simulink library "aerolib_blown_block"  (R2022b)
settings: Solver=ode45  StartTime=0.0  StopTime=10.0  RelTol=1e-3
PostLoadFcn:
  | load_system('aerolibv1')
  | setsysloc('aerolibv1')
libraries: aerolibadynsys x6, sharedutil x1
Description:
  | Aerospace Blockset Library: Aerodynamic library
settings Model: FPTRunName=Active  Creator=The MathWorks, Inc.  LastModifiedBy=olinw
settings SolverCC: AlgebraicLoopSolver=TrustRegion  MaxZcPerStep=1
settings DataIOCC: LimitDataPoints=on  SaveFormat=Array  SignalLoggingSaveFormat=ModelDataLogs  ReturnWorkspaceOutputs=off
settings OptimizationCC: BlockReduction=off  BooleanDataType=off  ExpressionDepthLimit=2147483647  EfficientMapNaN2IntZero=off  LifeSpan=inf
settings DebuggingCC: SaveWithParameterizedLinksMsg=none  UnderspecifiedInitializationDetection=Classic  MergeDetectMultiDrivingBlocksExec=none  SignalResolutionControl=TryResolveAllWithWarning  FcnCallInpInsideContextMsg=warning  UnconnectedInputMsg=warning  UnconnectedOutputMsg=warning  UnconnectedLineMsg=warning  AllowSymbolicDim=off  StateNameClashWarn=warning  SFUnexpectedBacktrackingDiag=warning  SFNoUnconditionalDefaultTransitionDiag=warning  SFExecutionAtInitializationDiag=none  SFMachineParentedDataDiag=warning  ArithmeticOperatorsInVariantConditions=warning
settings HardwareCC: ProdBitPerPointer=32  ProdLargestAtomicFloat=None  ProdIntDivRoundTo=Undefined  ProdEndianess=Unspecified  ProdWordSize=32  ProdHWDeviceType=32-bit Generic  TargetUnknown=on
settings ModelReferenceCC: EnableRefExpFcnMdlSchedulingChecks=on  PropagateSignalLabelsOutOfModel=off
settings SFSimCC: SimUseLocalCustomCode=off  CustomCodeUndefinedFunction=UseInterfaceOnly
settings RTWCC: RTWUseLocalCustomCode=off  DLArmComputeVersion=19.05
settings CodeAppCC: StateflowObjectComments=on
settings GRTTargetCC: TargetLangStandard=C89/C90 (ANSI)  CombineOutputUpdateFcns=off  GRTInterface=on
settings ConfigComp: CovMetricSettings=dw  CovSaveCumulativeToWorkspaceVar=on  CovSaveSingleToWorkspaceVar=on  CovExternalEMLEnable=off

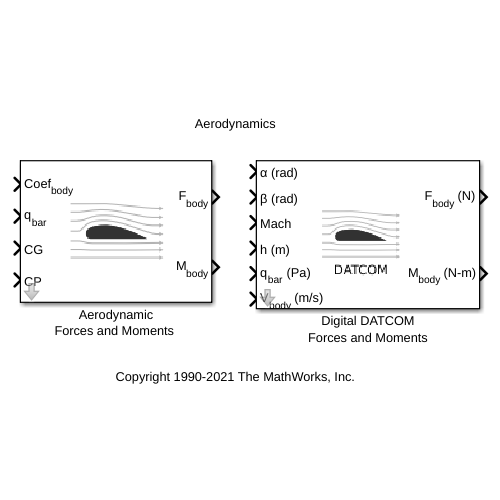
[thumbnail: Simulink's stored preview of the top-level diagram]
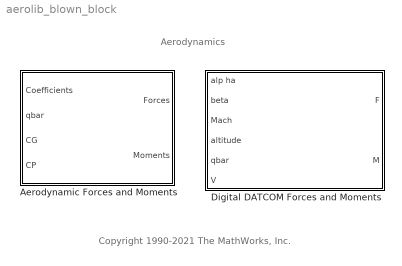
== system aerolib_blown_block ==
  note: Aerodynamics
  note: Copyright 1990-2021 The MathWorks, Inc.
  "Aerodynamic Forces and Moments " : Subsystem  BlockKeywords=__PRM__SERIALIZED__DATA__:Aerodynamic Forces and Moments,aerodynamics,aerodynamic coefficients  mask(Aerodynamic Forces and Moments){inputAxes=Body, outputForceAxes=Body, outputMomentAxes=Body, S=1, b=1, cbar=1}
      mask prompts: inputAxes "aeroblks:aeroblkadyn:blockAerodynamicForcesandMomentsParamInputaxes"; outputForceAxes "aeroblks:aeroblkadyn:blockAerodynamicForcesandMomentsParamForceaxes"; outputMomentAxes "aeroblks:aeroblkadyn:blockAerodynamicForcesandMomentsParamMomentaxes"; S "aeroblks:aeroblkadyn:blockAerodynamicForcesandMomentsParamReferencearea"; b "aeroblks:aeroblkadyn:blockAerodynamicForcesandMomentsParamReferencespan"; cbar "aeroblks:aeroblkadyn:blockAerodynamicForcesandMomentsParamReferencelength"
      mask help: aeroblks:aeroblkadyn:blockAerodynamicForcesandMomentsDesc
      mask init:
      | ports=aeroicon('aeroblkadyn','icon');
      mask Help: eval('asbhelp');
      mask TypeOptions inputAxes: aeroblks:aeroblkadyn:blockAerodynamicForcesandMomentsParamComboBody | aeroblks:aeroblkadyn:blockAerodynamicForcesandMomentsParamComboStability | aeroblks:aeroblkadyn:blockAerodynamicForcesandMomentsParamComboWind
      mask TypeOptions outputForceAxes: aeroblks:aeroblkadyn:blockAerodynamicForcesandMomentsParamComboBody | aeroblks:aeroblkadyn:blockAerodynamicForcesandMomentsParamComboStability | aeroblks:aeroblkadyn:blockAerodynamicForcesandMomentsParamComboWind
      mask TypeOptions outputMomentAxes: aeroblks:aeroblkadyn:blockAerodynamicForcesandMomentsParamComboBody | aeroblks:aeroblkadyn:blockAerodynamicForcesandMomentsParamComboStability | aeroblks:aeroblkadyn:blockAerodynamicForcesandMomentsParamComboWind
      mask DialogControl inputAxes Prompt: Input axes:
      mask DialogControl outputForceAxes Prompt: Force axes:
      mask DialogControl outputMomentAxes Prompt: Moment axes:
      mask DialogControl S Prompt: Reference area:
      mask DialogControl b Prompt: Reference span:
      mask DialogControl cbar Prompt: Reference length:
      mask Display:
      | port_label(ports(1).type,ports(1).port,ports(1).txt,'texmode','on');
      | port_label(ports(2).type,ports(2).port,ports(2).txt,'texmode','on');
      | port_label(ports(3).type,ports(3).port,ports(3).txt,'texmode','on');
      | port_label(ports(4).type,ports(4).port,ports(4).txt,'texmode','on');
      | port_label(ports(5).type,ports(5).port,ports(5).txt,'texmode','on');
      | port_label(ports(6).type,ports(6).port,ports(6).txt,'texmode','on');
      | port_label(ports(7).type,ports(7).port,ports(7).txt,'texmode','on');
  Digital DATCOM Forces and Moments : Subsystem  BlockKeywords=__PRM__SERIALIZED__DATA__:Digital DATCOM Forces and Moments,aerodynamics,aerodynamic coefficients,Airforce,Air Force,stability and control,USAF,DATCOM  mask(Digital DATCOM Forces and Moments){units=Metric (MKS), dcase=factstruct{1}, fmode=Body, buildno=0, imethod=None - flat, emethod=None - clip, rmethod=Clip to Range, action=None}
      mask prompts: units "aeroblks:aeroblkadyn:blockDigitalDATCOMForcesandMomentsParamUnits"; dcase "aeroblks:aeroblkadyn:blockDigitalDATCOMForcesandMomentsParamDigitalDATCOMstructure"; fmode "aeroblks:aeroblkadyn:blockDigitalDATCOMForcesandMomentsParamForceaxes"; buildno "aeroblks:aeroblkadyn:blockDigitalDATCOMForcesandMomentsParamBuildcase"; imethod "aeroblks:aeroblkadyn:blockDigitalDATCOMForcesandMomentsParamInterpolationmethod"; emethod "aeroblks:aeroblkadyn:blockDigitalDATCOMForcesandMomentsParamExtrapolationmethod"; rmethod "aeroblks:aeroblkadyn:blockDigitalDATCOMForcesandMomentsParamProcessoutofrangeinput"; action "aeroblks:aeroblkadyn:blockDigitalDATCOMForcesandMomentsParamActionforoutofrangeinput"
      mask help: aeroblks:aeroblkadyn:blockDigitalDATCOMForcesandMomentsDesc
      mask init:
      | dcase_str = dcase;
      | try
      |     dcase = slResolve(dcase,gcb);
      | catch
      |     dcase = struct('Invalid',true);
      | end
      | 
      | [ports]=aeroicon('aeroblkddatcom',dcase, dcase_str);
      mask Help: eval('asbhelp');
      mask TypeOptions units: aeroblks:aeroblkadyn:blockDigitalDATCOMForcesandMomentsParamComboMetricMKS | aeroblks:aeroblkadyn:blockDigitalDATCOMForcesandMomentsParamComboEnglishVelocityinfts | aeroblks:aeroblkadyn:blockDigitalDATCOMForcesandMomentsParamComboEnglishVelocityinkts
      mask TypeOptions fmode: aeroblks:aeroblkadyn:blockDigitalDATCOMForcesandMomentsParamComboBody | aeroblks:aeroblkadyn:blockDigitalDATCOMForcesandMomentsParamComboWind
      mask TypeOptions imethod: aeroblks:aeroblkadyn:blockDigitalDATCOMForcesandMomentsParamComboNoneflat | aeroblks:aeroblkadyn:blockDigitalDATCOMForcesandMomentsParamComboLinear
      mask TypeOptions emethod: aeroblks:aeroblkadyn:blockDigitalDATCOMForcesandMomentsParamComboNoneclip | aeroblks:aeroblkadyn:blockDigitalDATCOMForcesandMomentsParamComboLinear
      mask TypeOptions rmethod: aeroblks:aeroblkadyn:blockDigitalDATCOMForcesandMomentsParamComboCliptoRange | aeroblks:aeroblkadyn:blockDigitalDATCOMForcesandMomentsParamComboLinearExtrapolation
      mask TypeOptions action: aeroblks:aeroblkadyn:blockDigitalDATCOMForcesandMomentsParamComboNone | aeroblks:aeroblkadyn:blockDigitalDATCOMForcesandMomentsParamComboWarning | aeroblks:aeroblkadyn:blockDigitalDATCOMForcesandMomentsParamComboError
      mask Display:
      | port_label(ports(1).type,ports(1).port,ports(1).txt,'texmode','on');
      | port_label(ports(2).type,ports(2).port,ports(2).txt,'texmode','on');
      | port_label(ports(3).type,ports(3).port,ports(3).txt,'texmode','on');
      | port_label(ports(4).type,ports(4).port,ports(4).txt,'texmode','on');
      | port_label(ports(5).type,ports(5).port,ports(5).txt,'texmode','on');
      | port_label(ports(6).type,ports(6).port,ports(6).txt,'texmode','on');
      | port_label(ports(7).type,ports(7).port,ports(7).txt,'texmode','on');
      | port_label(ports(8).type,ports(8).port,ports(8).txt,'texmode','on');
      | port_label(ports(9).type,ports(9).port,ports(9).txt,'texmode','on');
      | port_label(ports(10).type,ports(10).port,ports(10).txt,'texmode','on');
      | port_label(ports(11).type,ports(11).port,ports(11).txt,'texmode','on');
      | port_label(ports(12).type,ports(12).port,ports(12).txt,'texmode','on');

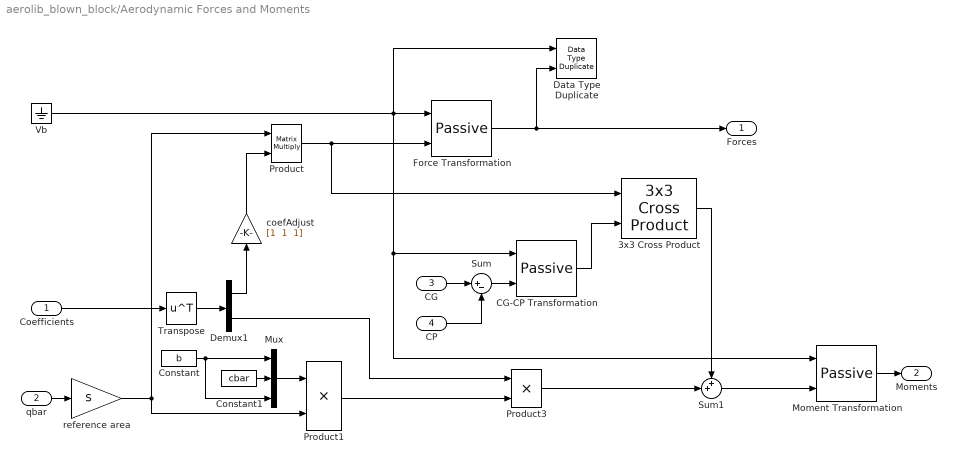
== system aerolib_blown_block/Aerodynamic Forces and Moments  ==
  Coefficients : Inport
  qbar : Inport  Port=2
  CG : Inport  Port=3
  CP : Inport  Port=4
  3x3 Cross Product : sharedutil/3x3 Cross Product  aMode=aMode
  CG-CP Transformation : aerolibadynsys/Passive  SystemSampleTime=-1  VariantActivationTime=update diagram  Latency=0  AutoFrameSizeCalculation=off
  Constant : Constant  Value=b
  Constant1 : Constant  Value=cbar
  Data Type Duplicate : DataTypeDuplicate
  Demux1 : Demux  Outputs=[3,3]
      settings: DisplayOption=none
  Force Transformation : aerolibadynsys/Passive  SystemSampleTime=-1  VariantActivationTime=update diagram  Latency=0  AutoFrameSizeCalculation=off
  Moment Transformation : aerolibadynsys/Passive  SystemSampleTime=-1  VariantActivationTime=update diagram  Latency=0  AutoFrameSizeCalculation=off
  Mux : Mux  Inputs=3
  Product : Product  Multiplication=Matrix(*)  InputSameDT=on  OutDataTypeStr=Inherit: Inherit via back propagation  SaturateOnIntegerOverflow=on
  Product1 : Product  OutDataTypeStr=Inherit: Inherit via back propagation  SaturateOnIntegerOverflow=on
  Product3 : Product  InputSameDT=on  SaturateOnIntegerOverflow=on  OutDataTypeStr=Inherit: Same as first input
  Sum : Sum  Inputs=|+-  InputSameDT=on  SaturateOnIntegerOverflow=on  OutDataTypeStr=Inherit: Same as first input
  Sum1 : Sum  Inputs=++|  InputSameDT=on  SaturateOnIntegerOverflow=on  OutDataTypeStr=Inherit: Same as first input
  Transpose : Math  Operator=transpose
  Vb : Ground
  coefAdjust : Gain  Gain="[1  1  1]"
  reference area : Gain  Gain=S  SaturateOnIntegerOverflow=on  OutDataTypeStr=Inherit: Same as input  ParamDataTypeStr=Inherit: Same as input
  Forces : Outport  VectorParamsAs1DForOutWhenUnconnected=off
  Moments : Outport  Port=2  VectorParamsAs1DForOutWhenUnconnected=off
  wires:
  CG-CP Transformation/1 -> 3x3 Cross Product/2
  Sum/1 -> CG-CP Transformation/2
  CP/1 -> Sum/2
  CG/1 -> Sum/1
  coefAdjust/1 -> Product/2
  Vb/1 -> Data Type Duplicate/1, Force Transformation/1, Moment Transformation/1, CG-CP Transformation/1
  Moment Transformation/1 -> Moments/1
  Sum1/1 -> Moment Transformation/2
  Force Transformation/1 -> Data Type Duplicate/2, Forces/1
  Product/1 -> 3x3 Cross Product/1, Force Transformation/2
  Demux1/1 -> coefAdjust/1
  Product3/1 -> Sum1/2
  reference area/1 -> Product/1, Product1/2
  qbar/1 -> reference area/1
  Demux1/2 -> Product3/1
  Coefficients/1 -> Transpose/1
  Product1/1 -> Product3/2
  3x3 Cross Product/1 -> Sum1/1
  Constant1/1 -> Mux/2
  Constant/1 -> Mux/3, Mux/1
  Mux/1 -> Product1/1
  Transpose/1 -> Demux1/1

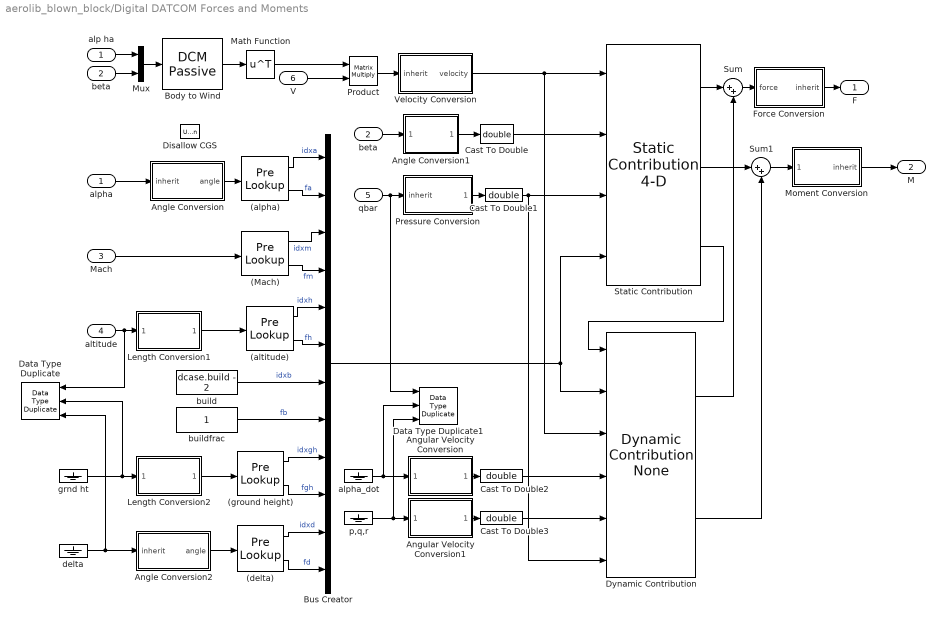
== system aerolib_blown_block/Digital DATCOM Forces and Moments ==
  alp ha : Inport  Unit=rad
  beta : Inport  Port=2  Unit=rad
  Mach : Inport  Port=3  Unit=1
  altitude : Inport  Port=4  Unit=m
  qbar : Inport  Port=5  Unit=Pa
  V : Inport  Port=6  Unit=m/s
  (Mach) : PreLookup  BreakpointsData=0:2  BeginIndexSearchUsingPreviousIndexResult=on  IndexDataTypeStr=int32  FractionDataTypeStr=double
  (alpha) : PreLookup  BreakpointsData=dcase.alpha  BeginIndexSearchUsingPreviousIndexResult=on  IndexDataTypeStr=int32  FractionDataTypeStr=double
  (altitude) : PreLookup  BreakpointsData=0:2  BeginIndexSearchUsingPreviousIndexResult=on  IndexDataTypeStr=int32  FractionDataTypeStr=double
  (delta) : PreLookup  BreakpointsData=[0:2]  BeginIndexSearchUsingPreviousIndexResult=on  IndexDataTypeStr=int32  FractionDataTypeStr=double
  (ground height) : PreLookup  BreakpointsData=[0:2]  BeginIndexSearchUsingPreviousIndexResult=on  IndexDataTypeStr=int32  FractionDataTypeStr=double
  Angle Conversion : Subsystem
  Angle Conversion1 : Subsystem
  Angle Conversion2 : Subsystem
  Angular Velocity Conversion : Subsystem
  Angular Velocity Conversion1 : Subsystem
  Body to Wind : aerolibadynsys/DCM Passive  SystemSampleTime=-1  VariantActivationTime=update diagram  Latency=0  AutoFrameSizeCalculation=off
  Bus Creator : BusCreator  Inputs=12
  Cast To Double{,1..3} (4 alike) : DataTypeConversion  OutDataTypeStr=double  SaturateOnIntegerOverflow=off  RndMeth=Floor
  Data Type Duplicate : DataTypeDuplicate  NumInputPorts=3
  Data Type Duplicate1 : DataTypeDuplicate  NumInputPorts=3
  Disallow CGS : UnitConfiguration  UnitSystemsStr=English,SI,SI (extended)  AllowAllUnitSystems=off
  Dynamic Contribution : aerolibadynsys/Dynamic Contribution None  Unit=deg/s
  Force Conversion : Subsystem
  Length Conversion1 : Subsystem
  Length Conversion2 : Subsystem
  Math Function : Math  Operator=transpose  SignedPower=on
  Moment Conversion : Subsystem
  Mux : Mux  Inputs=2
  Pressure Conversion : Subsystem
  Product : Product  Multiplication=Matrix(*)  InputSameDT=on  RndMeth=Zero
  Static Contribution : aerolibadynsys/Static Contribution 4-D  SystemSampleTime=-1  VariantActivationTime=update diagram  Latency=0  AutoFrameSizeCalculation=off
  Sum : Sum  Inputs=|++
  Sum1 : Sum  Inputs=|++
  Velocity Conversion : Subsystem
  alpha : InportShadow  Unit=rad
  alpha_dot : Ground
  "beta " : InportShadow  Port=2  Unit=rad
  build : Constant  Value=dcase.build - 2  OutDataTypeStr=int32
  buildfrac : Constant  OutDataTypeStr=double
  delta : Ground
  grnd ht : Ground
  p,q,r : Ground
  F : Outport  Unit=N  VectorParamsAs1DForOutWhenUnconnected=off
  M : Outport  Port=2  Unit=N*m  VectorParamsAs1DForOutWhenUnconnected=off
  wires:
  V/1 -> Product/2
  Math Function/1 -> Product/1
  "beta "/1 -> Mux/2
  alp ha/1 -> Mux/1
  Mux/1 -> Body to Wind/1
  Body to Wind/1 -> Math Function/1
  Bus Creator/1 -> Dynamic Contribution/2, Static Contribution/4
  Angle Conversion2/1(angle) -> (delta)/1
  (alpha)/1 -> Bus Creator/1  "idxa"
  (Mach)/1 -> Bus Creator/3  "idxm"
  Mach/1 -> (Mach)/1
  alpha/1 -> Angle Conversion/1(inherit)
  altitude/1 -> Data Type Duplicate/1, Length Conversion1/1(inherit)
  Sum/1 -> Force Conversion/1(force)
  p,q,r/1 -> Data Type Duplicate1/3, Angular Velocity Conversion1/1(inherit)
  delta/1 -> Angle Conversion2/1(inherit), Data Type Duplicate/3
  Static Contribution/3 -> Dynamic Contribution/1
  beta/1 -> Angle Conversion1/1(inherit)
  Product/1 -> Velocity Conversion/1(inherit)
  qbar/1 -> Data Type Duplicate1/1, Pressure Conversion/1(inherit)
  Static Contribution/1 -> Sum/1
  Dynamic Contribution/1 -> Sum/2
  Static Contribution/2 -> Sum1/1
  Dynamic Contribution/2 -> Sum1/2
  alpha_dot/1 -> Angular Velocity Conversion/1(inherit), Data Type Duplicate1/2
  grnd ht/1 -> Data Type Duplicate/2, Length Conversion2/1(inherit)
  Force Conversion/1(inherit) -> F/1
  Moment Conversion/1(inherit) -> M/1
  Angular Velocity Conversion/1(velocity) -> Cast To Double2/1
  Angular Velocity Conversion1/1(velocity) -> Cast To Double3/1
  Velocity Conversion/1(velocity) -> Dynamic Contribution/3, Static Contribution/1
  Pressure Conversion/1(pressure) -> Cast To Double1/1
  Length Conversion1/1(length) -> (altitude)/1
  Length Conversion2/1(length) -> (ground height)/1
  (delta)/1 -> Bus Creator/11  "idxd"
  (delta)/2 -> Bus Creator/12  "fd"
  (ground height)/1 -> Bus Creator/9  "idxgh"
  (ground height)/2 -> Bus Creator/10  "fgh"
  build/1 -> Bus Creator/7  "idxb"
  buildfrac/1 -> Bus Creator/8  "fb"
  (altitude)/1 -> Bus Creator/5  "idxh"
  (altitude)/2 -> Bus Creator/6  "fh"
  (Mach)/2 -> Bus Creator/4  "fm"
  (alpha)/2 -> Bus Creator/2  "fa"
  Angle Conversion/1(angle) -> (alpha)/1
  Angle Conversion1/1(angle) -> Cast To Double/1
  Sum1/1 -> Moment Conversion/1(moment)
  Cast To Double/1 -> Static Contribution/2
  Cast To Double1/1 -> Static Contribution/3, Dynamic Contribution/6
  Cast To Double2/1 -> Dynamic Contribution/4
  Cast To Double3/1 -> Dynamic Contribution/5

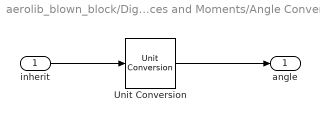
== system aerolib_blown_block/Digital DATCOM Forces and Moments/Angle Conversion ==
  inherit : Inport
  Unit Conversion : UnitConversion
  angle : Outport  Unit=deg  VectorParamsAs1DForOutWhenUnconnected=off
  wires:
  Unit Conversion/1 -> angle/1
  inherit/1 -> Unit Conversion/1

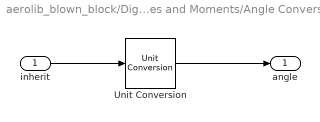
== system aerolib_blown_block/Digital DATCOM Forces and Moments/Angle Conversion1 ==
  inherit : Inport
  Unit Conversion : UnitConversion
  angle : Outport  Unit=deg  VectorParamsAs1DForOutWhenUnconnected=off
  wires:
  inherit/1 -> Unit Conversion/1
  Unit Conversion/1 -> angle/1

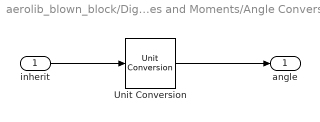
== system aerolib_blown_block/Digital DATCOM Forces and Moments/Angle Conversion2 ==
  inherit : Inport  Unit=rad
  Unit Conversion : UnitConversion
  angle : Outport  Unit=deg  VectorParamsAs1DForOutWhenUnconnected=off
  wires:
  inherit/1 -> Unit Conversion/1
  Unit Conversion/1 -> angle/1

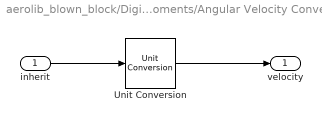
== system aerolib_blown_block/Digital DATCOM Forces and Moments/Angular Velocity Conversion ==
  inherit : Inport  Unit=rad/s
  Unit Conversion : UnitConversion
  velocity : Outport  Unit=deg/s  VectorParamsAs1DForOutWhenUnconnected=off
  wires:
  inherit/1 -> Unit Conversion/1
  Unit Conversion/1 -> velocity/1

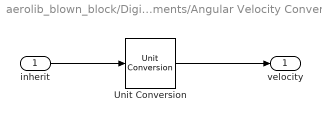
== system aerolib_blown_block/Digital DATCOM Forces and Moments/Angular Velocity Conversion1 ==
  inherit : Inport  Unit=rad/s
  Unit Conversion : UnitConversion
  velocity : Outport  Unit=deg/s  VectorParamsAs1DForOutWhenUnconnected=off
  wires:
  Unit Conversion/1 -> velocity/1
  inherit/1 -> Unit Conversion/1

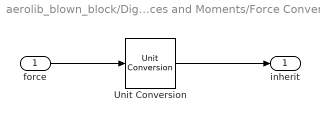
== system aerolib_blown_block/Digital DATCOM Forces and Moments/Force Conversion ==
  force : Inport  Unit=lbf
  Unit Conversion : UnitConversion  OutputType=Inherit: Inherit via back propagation
  inherit : Outport  VectorParamsAs1DForOutWhenUnconnected=off
  wires:
  Unit Conversion/1 -> inherit/1
  force/1 -> Unit Conversion/1

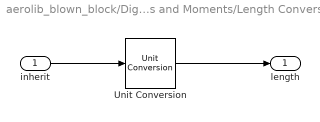
== system aerolib_blown_block/Digital DATCOM Forces and Moments/Length Conversion1 ==
  inherit : Inport
  Unit Conversion : UnitConversion
  length : Outport  Unit=ft  VectorParamsAs1DForOutWhenUnconnected=off
  wires:
  Unit Conversion/1 -> length/1
  inherit/1 -> Unit Conversion/1

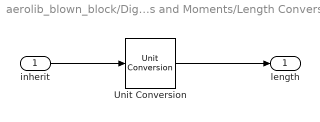
== system aerolib_blown_block/Digital DATCOM Forces and Moments/Length Conversion2 ==
  inherit : Inport  Unit=m
  Unit Conversion : UnitConversion
  length : Outport  Unit=ft  VectorParamsAs1DForOutWhenUnconnected=off
  wires:
  inherit/1 -> Unit Conversion/1
  Unit Conversion/1 -> length/1

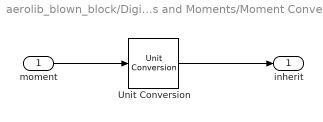
== system aerolib_blown_block/Digital DATCOM Forces and Moments/Moment Conversion ==
  moment : Inport  Unit=lbf*ft
  Unit Conversion : UnitConversion  OutputType=Inherit: Inherit via back propagation
  inherit : Outport  VectorParamsAs1DForOutWhenUnconnected=off
  wires:
  Unit Conversion/1 -> inherit/1
  moment/1 -> Unit Conversion/1

== system aerolib_blown_block/Digital DATCOM Forces and Moments/Pressure Conversion ==
  inherit : Inport
  Unit Conversion : UnitConversion
  pressure : Outport  Unit=lbf/ft^2  VectorParamsAs1DForOutWhenUnconnected=off
  wires:
  inherit/1 -> Unit Conversion/1
  Unit Conversion/1 -> pressure/1

== system aerolib_blown_block/Digital DATCOM Forces and Moments/Velocity Conversion ==
  inherit : Inport  Unit=m/s
  Unit Conversion : UnitConversion  OutputType=Inherit: Inherit via back propagation
  velocity : Outport  Unit=ft/s  VectorParamsAs1DForOutWhenUnconnected=off
  wires:
  Unit Conversion/1 -> velocity/1
  inherit/1 -> Unit Conversion/1
